simulink model "SecRwLtStZeroIsPosChk"  (R2018b)
settings: Solver=FixedStepDiscrete  StartTime=0.0  StopTime=10.0  RelTol=1e-3
undefined symbols (not defined in the file or in its folder): KeSMSuSecRwStZeroPosDelta_Val, KeSMSuSecRwStZeroPosTolr_Val
settings Model: ModifiedHistory=2024.7.8 V3.0.0 557模式流程V1.9  Creator=sn2xws  LastModifiedBy=sn2xws
settings DataIOCC: SaveFormat=StructureWithTime
settings OptimizationCC: DefaultParameterBehavior=Inlined  EnhancedBackFolding=on  PassReuseOutputArgsAs=Individual arguments  ZeroExternalMemoryAtStartup=off  ZeroInternalMemoryAtStartup=off  OptimizeBlockOrder=speed  DifferentSizesBufferReuse=on  OptimizationCustomize=off
settings DebuggingCC: ParameterTunabilityLossMsg=error
settings SFSimCC: MATLABDynamicMemAlloc=off
settings RTWCC: SystemTargetFile=autosar.tlc  GenCodeOnly=on  TemplateMakefile=ert_default_tmf  Description=AUTOSAR  GenerateReport=on  IncludeHyperlinkInReport=on  LaunchReport=on  GenerateTraceInfo=on  GenerateTraceReport=on  GenerateTraceReportSl=on  GenerateTraceReportSf=on  GenerateTraceReportEml=on
settings CodeAppCC: ForceParamTrailComments=on  IgnoreCustomStorageClasses=off  OperatorAnnotations=on  SimulinkDataObjDesc=on  SFDataObjDesc=on  InsertBlockDesc=on
settings STFCustomTargetCC: TargetLangStandard=C99 (ISO)  MultiwordLength=256  ParMdlRefBuildCompliant=on  CompOptLevelCompliant=on  IncludeMdlTerminateFcn=off  CombineOutputUpdateFcns=on  SuppressErrorStatus=on  ERTCustomFileBanners=on  SupportNonFinite=off  SupportComplex=off  SupportContinuousTime=off  SupportNonInlinedSFcns=off  RemoveResetFunc=on  MATLABClassNameForMDSCustomization=Simulink.SoftwareTarget.ERTCustomization  AutosarCompliant=on  UseToolchainInfoCompliant=on  LookupTableObjectStructAxisOrder=2,1,3,4,...  LUTObjectStructOrderEvenSpacing=Size,Table,Breakpoints  SystemTargetFile=autosar.tlc
settings ERTTargetCC: TargetLangStandard=C99 (ISO)  ConcurrentExecutionCompliant=off  IncludeMdlTerminateFcn=off  SuppressErrorStatus=on  SupportNonFinite=off  SupportComplex=off  ModelStepFunctionPrototypeControlCompliant=off  CPPClassGenCompliant=off  AutosarCompliant=on  LookupTableObjectStructAxisOrder=2,1,3,4,...  LUTObjectStructOrderEvenSpacing=Size,Table,Breakpoints  InlinedParameterPlacement=NonHierarchical  ERTCustomFileTemplate=example_file_process.tlc  ERTFilePackagingFormat=Compact

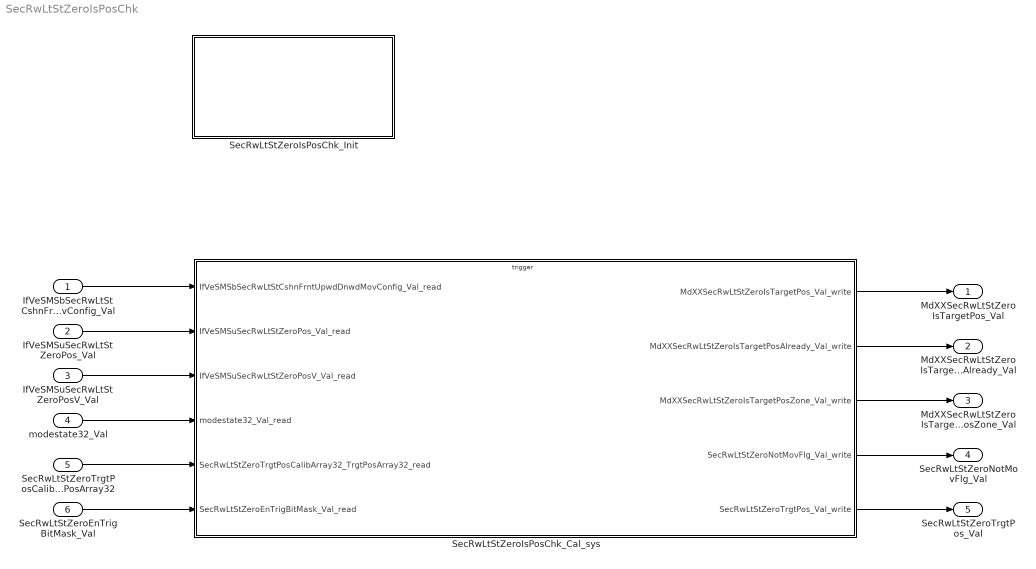
== system SecRwLtStZeroIsPosChk ==
  IfVeSMSbSecRwLtStCshnFrntUpwdDnwdMovConfig_Val : Inport  OutDataTypeStr=boolean  PortDimensions=1
  IfVeSMSuSecRwLtStZeroPos_Val : Inport  Port=2  OutDataTypeStr=uint16  PortDimensions=1
  IfVeSMSuSecRwLtStZeroPosV_Val : Inport  Port=3  OutDataTypeStr=boolean  PortDimensions=1
  modestate32_Val : Inport  Port=4  OutDataTypeStr=uint32  PortDimensions=1
  SecRwLtStZeroTrgtPosCalibArray32_TrgtPosArray32 : Inport  Description=|  Port=5  OutDataTypeStr=uint16  PortDimensions=96
      | 0:Pos
      | 1:Max
      | 2:Min
  SecRwLtStZeroEnTrigBitMask_Val : Inport  Port=6  OutDataTypeStr=uint32  PortDimensions=1
  SecRwLtStZeroIsPosChk_Cal_sys : Subsystem
  SecRwLtStZeroIsPosChk_Init : Subsystem
  MdXXSecRwLtStZeroIsTargetPos_Val : Outport  OutDataTypeStr=uint32  PortDimensions=1
  MdXXSecRwLtStZeroIsTargetPosAlready_Val : Outport  Port=2  OutDataTypeStr=uint32  PortDimensions=1
  MdXXSecRwLtStZeroIsTargetPosZone_Val : Outport  Port=3  OutDataTypeStr=uint32  PortDimensions=1
  SecRwLtStZeroNotMovFlg_Val : Outport  Port=4  OutDataTypeStr=boolean  PortDimensions=1
  SecRwLtStZeroTrgtPos_Val : Outport  Port=5  OutDataTypeStr=uint16  PortDimensions=1
  wires:
  IfVeSMSbSecRwLtStCshnFrntUpwdDnwdMovConfig_Val/1 -> SecRwLtStZeroIsPosChk_Cal_sys/1(IfVeSMSbSecRwLtStCshnFrntUpwdDnwdMovConfig_Val_read)
  IfVeSMSuSecRwLtStZeroPos_Val/1 -> SecRwLtStZeroIsPosChk_Cal_sys/2(IfVeSMSuSecRwLtStZeroPos_Val_read)
  IfVeSMSuSecRwLtStZeroPosV_Val/1 -> SecRwLtStZeroIsPosChk_Cal_sys/3(IfVeSMSuSecRwLtStZeroPosV_Val_read)
  modestate32_Val/1 -> SecRwLtStZeroIsPosChk_Cal_sys/4(modestate32_Val_read)
  SecRwLtStZeroIsPosChk_Cal_sys/1(MdXXSecRwLtStZeroIsTargetPos_Val_write) -> MdXXSecRwLtStZeroIsTargetPos_Val/1
  SecRwLtStZeroIsPosChk_Cal_sys/2(MdXXSecRwLtStZeroIsTargetPosAlready_Val_write) -> MdXXSecRwLtStZeroIsTargetPosAlready_Val/1
  SecRwLtStZeroIsPosChk_Cal_sys/3(MdXXSecRwLtStZeroIsTargetPosZone_Val_write) -> MdXXSecRwLtStZeroIsTargetPosZone_Val/1
  SecRwLtStZeroIsPosChk_Cal_sys/4(SecRwLtStZeroNotMovFlg_Val_write) -> SecRwLtStZeroNotMovFlg_Val/1
  SecRwLtStZeroIsPosChk_Cal_sys/5(SecRwLtStZeroTrgtPos_Val_write) -> SecRwLtStZeroTrgtPos_Val/1
  SecRwLtStZeroTrgtPosCalibArray32_TrgtPosArray32/1 -> SecRwLtStZeroIsPosChk_Cal_sys/5(SecRwLtStZeroTrgtPosCalibArray32_TrgtPosArray32_read)
  SecRwLtStZeroEnTrigBitMask_Val/1 -> SecRwLtStZeroIsPosChk_Cal_sys/6(SecRwLtStZeroEnTrigBitMask_Val_read)

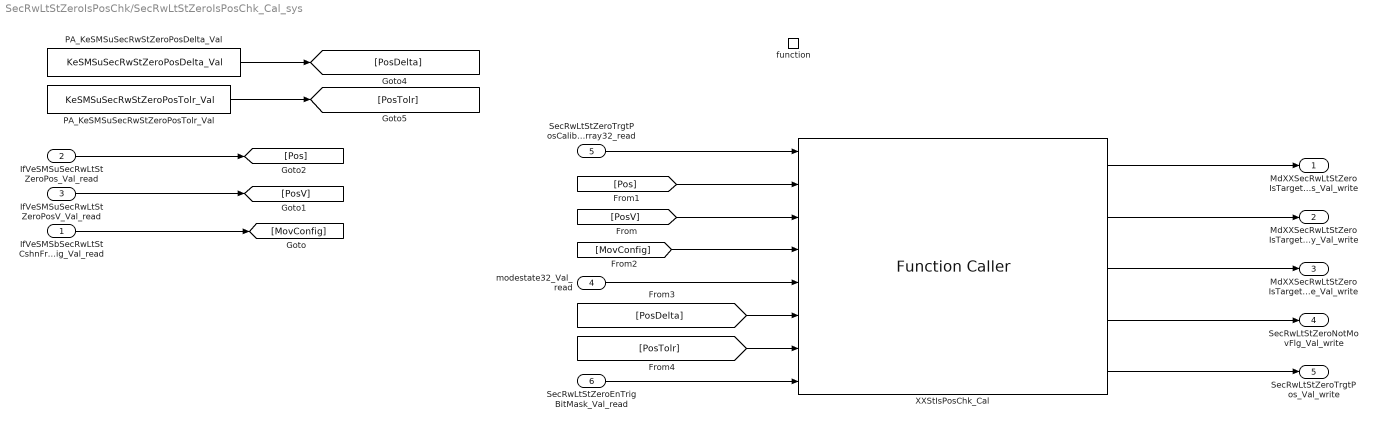
== system SecRwLtStZeroIsPosChk/SecRwLtStZeroIsPosChk_Cal_sys ==
  IfVeSMSbSecRwLtStCshnFrntUpwdDnwdMovConfig_Val_read : Inport
  IfVeSMSuSecRwLtStZeroPos_Val_read : Inport  Port=2
  IfVeSMSuSecRwLtStZeroPosV_Val_read : Inport  Port=3
  modestate32_Val_read : Inport  Port=4
  SecRwLtStZeroTrgtPosCalibArray32_TrgtPosArray32_read : Inport  Port=5
  SecRwLtStZeroEnTrigBitMask_Val_read : Inport  Port=6
  function : TriggerPort  TriggerType=function-call  IsSimulinkFunction=on  FunctionName=SecRwLtStZeroIsPosChk_Cal  VariantControl=(inherit)
  PA_KeSMSuSecRwStZeroPosDelta_Val : Constant  Value=KeSMSuSecRwStZeroPosDelta_Val
  PA_KeSMSuSecRwStZeroPosTolr_Val : Constant  Value=KeSMSuSecRwStZeroPosTolr_Val
  XXStIsPosChk_Cal : FunctionCaller  FunctionPrototype=[IsPos,IsPosAlready,IsPosZone,NotMovFlg,StTrgtPos] = XXStIsPosChk_Cal(MdCalibArray32,Pos,PosV,MovConfig,modestate32,PosDelta,PosTolr,StBitMask)  InputArgumentSpecifications=uint16([1;1;1;1;1;1;1;1;1;1;1;1;1;1;1;1;1;1;1;1;1;1;1;1;1;1;1;1;1;1;1;1;1;1;1;1;1;1;1;1;1;1;1;1;1;1;1;1;1;1;1;1;1;1;1;1;1;1;1;1;1;1;1;1;1;1;1;1;1;1;1;1;1;1;1;1;1;1;1;1;1;1;1;1;1;1;1;1;1;1;1;1;1;1;1;1]), uint16(1), boolean(true), boolean(true), uint32(1), uint16(1), uint16(1), uint32(1)  OutputArgumentSpecifications=uint32(1), uint32(1), uint32(1), boolean(true), uint16(1)
  MdXXSecRwLtStZeroIsTargetPos_Val_write : Outport
      settings: EnsureOutportIsVirtual=on
  MdXXSecRwLtStZeroIsTargetPosAlready_Val_write : Outport  Port=2
      settings: EnsureOutportIsVirtual=on
  MdXXSecRwLtStZeroIsTargetPosZone_Val_write : Outport  Port=3
      settings: EnsureOutportIsVirtual=on
  SecRwLtStZeroNotMovFlg_Val_write : Outport  Port=4
      settings: EnsureOutportIsVirtual=on
  SecRwLtStZeroTrgtPos_Val_write : Outport  Port=5
      settings: EnsureOutportIsVirtual=on
  wires:
  IfVeSMSbSecRwLtStCshnFrntUpwdDnwdMovConfig_Val_read/1 -> [MovConfig]
  IfVeSMSuSecRwLtStZeroPos_Val_read/1 -> [Pos]
  IfVeSMSuSecRwLtStZeroPosV_Val_read/1 -> [PosV]
  PA_KeSMSuSecRwStZeroPosDelta_Val/1 -> [PosDelta]
  PA_KeSMSuSecRwStZeroPosTolr_Val/1 -> [PosTolr]
  [PosV] -> XXStIsPosChk_Cal/3
  [Pos] -> XXStIsPosChk_Cal/2
  XXStIsPosChk_Cal/5 -> SecRwLtStZeroTrgtPos_Val_write/1
  SecRwLtStZeroTrgtPosCalibArray32_TrgtPosArray32_read/1 -> XXStIsPosChk_Cal/1
  XXStIsPosChk_Cal/4 -> SecRwLtStZeroNotMovFlg_Val_write/1
  modestate32_Val_read/1 -> XXStIsPosChk_Cal/5
  XXStIsPosChk_Cal/1 -> MdXXSecRwLtStZeroIsTargetPos_Val_write/1
  XXStIsPosChk_Cal/2 -> MdXXSecRwLtStZeroIsTargetPosAlready_Val_write/1
  XXStIsPosChk_Cal/3 -> MdXXSecRwLtStZeroIsTargetPosZone_Val_write/1
  [MovConfig] -> XXStIsPosChk_Cal/4
  [PosDelta] -> XXStIsPosChk_Cal/6
  [PosTolr] -> XXStIsPosChk_Cal/7
  SecRwLtStZeroEnTrigBitMask_Val_read/1 -> XXStIsPosChk_Cal/8

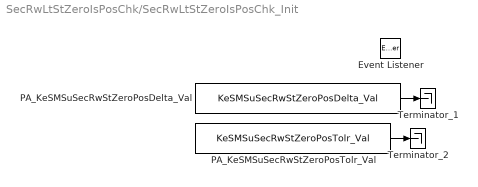
== system SecRwLtStZeroIsPosChk/SecRwLtStZeroIsPosChk_Init ==
  Event Listener : EventListener  EventName=reset
  PA_KeSMSuSecRwStZeroPosDelta_Val : Constant  Value=KeSMSuSecRwStZeroPosDelta_Val
  PA_KeSMSuSecRwStZeroPosTolr_Val : Constant  Value=KeSMSuSecRwStZeroPosTolr_Val
  Terminator_1 : Terminator
  Terminator_2 : Terminator
  wires:
  PA_KeSMSuSecRwStZeroPosDelta_Val/1 -> Terminator_1/1
  PA_KeSMSuSecRwStZeroPosTolr_Val/1 -> Terminator_2/1
